simulink model "sim_9"  (R2018a)
settings: Solver=VariableStepAuto  StartTime=0.0  StopTime=50  RelTol=1e-3
settings Model: Creator=Toshiba  LastModifiedBy=Toshiba
settings SolverCC: AlgebraicLoopSolver=LineSearch

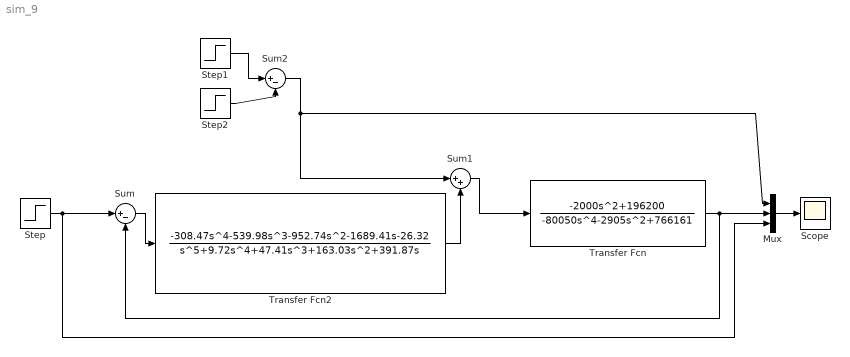
== system sim_9 ==
  Mux : Mux  Inputs=3
  Scope : Scope
  Step : Step  SampleTime=0
  Step1 : Step  Time=30  After=2  SampleTime=0
  Step2 : Step  Time=33  After=2  SampleTime=0
  Sum : Sum  Inputs=|+-
  Sum1 : Sum  Inputs=|++
  Sum2 : Sum  Inputs=|+-
  Transfer Fcn : TransferFcn  Numerator=[-2000, 0, 196200]  Denominator=[-80050, 0, -2905, 0, 766161]
  Transfer Fcn2 : TransferFcn  Numerator=[-308.47 -539.98 -952.74 -1689.41 -26.32]  Denominator=[1 9.72 47.41 163.03 391.87 0]
  wires:
  Step/1 -> Sum/1, Mux/3
  Sum/1 -> Transfer Fcn2/1
  Transfer Fcn/1 -> Sum/2, Mux/2
  Sum2/1 -> Sum1/1, Mux/1
  Transfer Fcn2/1 -> Sum1/2
  Sum1/1 -> Transfer Fcn/1
  Mux/1 -> Scope/1
  Step1/1 -> Sum2/1
  Step2/1 -> Sum2/2
